simulink library "Power_Shaft1_FuelCell_A1"  (R2025b)
settings: Solver=VariableStepAuto  StartTime=0.0  StopTime=10.0  RelTol=1e-3
undefined symbols (not defined in the file): Init, Powertrain
libraries: fl_lib x85, nesl_utility x30, GasN_lib x21, simulink_extras x6, SimscapeFluids_lib x6, customMath_lib x5, ee_lib x3, slpidlib x3, gn_supplement_lib x2, batteryecm_lib x1, simulink x1, sm_lib x1
(part 3 of 3)

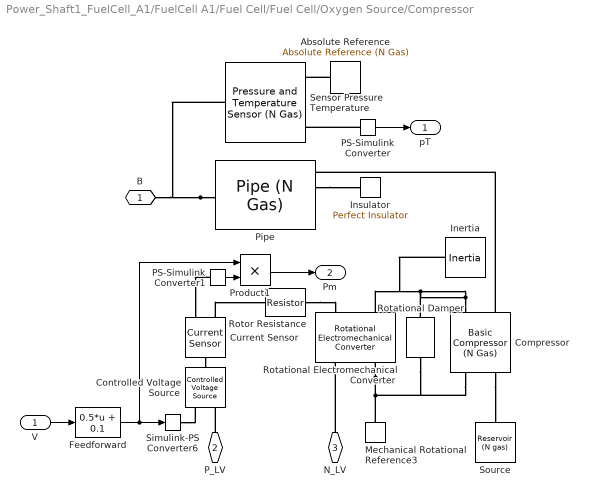
== system Power_Shaft1_FuelCell_A1/FuelCell A1/Fuel Cell/Fuel Cell/Oxygen Source/Compressor ==
  V : Inport
  Absolute Reference : GasN_lib/Absolute Reference (N Gas)
      settings: InternalSimscapePortConfiguration="{\"Bottom\":[],\"Left\":[{\"id\":\"A\",\"label\":\"\",\"type\":\"GasN.GasN\"}],\"Right\":[],\"Top\":[]}"
  Compressor : GasN_lib/Basic Compressor (N Gas)  pr_des=FuelCell.Compressor.rPressure.Value  mdot_corr_des=FuelCell.Compressor.mdotDesign.Value kg/s  omega_corr_des=FuelCell.Compressor.wDesign.Value rad/s  p_ref=FuelCell.Compressor.pReference.Value MPa  T_ref=FuelCell.Compressor.TReference.Value K  RH_ref=FuelCell.Compressor.relHumidity.Value  b1=FuelCell.Compressor.kSpeedCurve.Value  b2=FuelCell.Compressor.kSpeedOffset.Value  b3=FuelCell.Compressor.kSpeedSharp.Value  eta_poly=FuelCell.Compressor.effPolytropic.Value  eta_mech=FuelCell.Compressor.effMechanical.Value  area_A=FuelCell.Compressor.areaInlet.Value cm^2  area_B=FuelCell.Compressor.areaOutlet.Value cm^2  mdot_A_specify=off  mdot_A_priority=None  mdot_A=0.1 kg/s  mdot_A_nominal_specify=off  mdot_A_nominal_value=1  mdot_A_nominal_unit=kg/s  mdot_B_specify=off  mdot_B_priority=None  mdot_B=0.1 kg/s  mdot_B_nominal_specify=off  mdot_B_nominal_value=1  mdot_B_nominal_unit=kg/s  Phi_A_specify=off  Phi_A_priority=None  Phi_A=0 J/s  Phi_A_nominal_specify=off  Phi_A_nominal_value=1  Phi_A_nominal_unit=J/s  Phi_B_specify=off  Phi_B_priority=None  Phi_B=0 J/s  Phi_B_nominal_specify=off  Phi_B_nominal_value=1  Phi_B_nominal_unit=J/s  mdot_A_i_specify=off  mdot_A_i_priority=None  mdot_A_i=[ 0; 0; 0; 0 ] kg/s  mdot_A_i_nominal_specify=off  mdot_A_i_nominal_value=1  mdot_A_i_nominal_unit=kg/s  mdot_B_i_specify=off  mdot_B_i_priority=None  mdot_B_i=[ 0; 0; 0; 0 ] kg/s  mdot_B_i_nominal_specify=off  mdot_B_i_nominal_value=1  mdot_B_i_nominal_unit=kg/s  torque_specify=off  torque_priority=None  torque=1 N*m  torque_nominal_specify=off  torque_nominal_value=1  torque_nominal_unit=N*m
      settings: InternalSimscapePortConfiguration="{\"Bottom\":[],\"Left\":[{\"id\":\"A\",\"label\":\"A\",\"type\":\"GasN.GasN\"},{\"id\":\"Case\",\"label\":\"C\",\"type\":\"foundation.mechanical.rotational.rotational\"}],\"Right\":[{\"id\":\"B\",\"label\":\"B\",\"type\":\"GasN.GasN\"},{\"id\":\"Rod\",\"label\":\"R\",\"type\":\"foundation.mechanical.rotational.rotational\"}],\"Top\":[]}"
  Controlled Voltage Source : fl_lib/Electrical/Electrical Sources/Controlled Voltage Source
  Current Sensor : fl_lib/Electrical/Electrical Sensors/Current Sensor
  Feedforward : Fcn  Expr=0.5*u + 0.1
  Inertia : fl_lib/Mechanical/Rotational Elements/Inertia  inertia=FuelCell.Compressor.J.Value kg*m^2  num_ports=foundation.enum.numPorts2.one  w_specify=on  w_priority=High  w=0 rad/s  w_nominal_specify=off  w_nominal_value=1  w_nominal_unit=rad/s  t_specify=off  t_priority=None  t=0 N*m  t_nominal_specify=off  t_nominal_value=1  t_nominal_unit=N*m
  Insulator : fl_lib/Thermal/Thermal Elements/Perfect Insulator  T_specify=off  T_priority=None  T=0 K  T_nominal_specify=off  T_nominal_value=1  T_nominal_unit=K
  Mechanical Rotational Reference3 : fl_lib/Mechanical/Rotational Elements/Mechanical Rotational Reference
  PS-Simulink Converter : nesl_utility/PS-Simulink Converter  PhysicalDomain=network_engine_domain  SubClassName=ps_output  LeftPortType=input  RightPortType=output  PseudoPeriodic=off  Frequencies=[]  VectorFormat=1-D array  Unit=Pa  AffineConversion=off
  PS-Simulink Converter1 : nesl_utility/PS-Simulink Converter  PhysicalDomain=network_engine_domain  SubClassName=ps_output  LeftPortType=input  RightPortType=output  PseudoPeriodic=off  Frequencies=[]  VectorFormat=1-D array  Unit=A  AffineConversion=off
  Pipe : GasN_lib/Pipe (N Gas)  length=FuelCell.CompressorPipe.xPipe.Value m  area=FuelCell.CompressorPipe.areaPipe.Value cm^2  Dh=FuelCell.CompressorPipe.dHydraulic.Value cm  extra_length=FuelCell.CompressorPipe.xFriction.Value m  roughness=FuelCell.CompressorPipe.roughness.Value m  Re_lam=FuelCell.CompressorPipe.laminarReynoldsMax.Value  Re_tur=FuelCell.CompressorPipe.turbulentReynoldsMin.Value  shape_factor=FuelCell.CompressorPipe.frictionDarcy.Value  Nu_lam=FuelCell.CompressorPipe.laminarNusselt.Value  p0=FuelCell.CompressorPipe.p.Value MPa  T0=FuelCell.CompressorPipe.T.Value degC  comp=GasN.composition_enum.mole  y0=FuelCell.CompressorPipe.rMoleFractions.Value'  x0=[1; 0; 0; 0]  tau_c=FuelCell.CompressorPipe.timeCondensation.Value s  isCond=FuelCell.CompressorPipe.speciesCondensed.Value'
      settings: InternalSimscapePortConfiguration="{\"Bottom\":[],\"Left\":[{\"id\":\"A\",\"label\":\"A\",\"type\":\"GasN.GasN\"},{\"id\":\"H\",\"label\":\"H\",\"type\":\"foundation.thermal.thermal\"},{\"id\":\"MIn\",\"label\":\"M_in\",\"type\":\"input\"},{\"id\":\"TIn\",\"label\":\"T_in\",\"type\":\"input\"}],\"Right\":[{\"id\":\"B\",\"label\":\"B\",\"type\":\"GasN.GasN\"}],\"Top\":[]}"
  Product1 : Product
  Rotational Electromechanical Converter : fl_lib/Electrical/Electrical Elements/Rotational Electromechanical Converter  K=FuelCell.Compressor.KMotor.Value V/(rad/s)  i_specify=off  i_priority=None  i=0 A  i_nominal_specify=off  i_nominal_value=1  i_nominal_unit=A  v_specify=off  v_priority=None  v=0 V  v_nominal_specify=off  v_nominal_value=1  v_nominal_unit=V  t_specify=off  t_priority=None  t=0 N*m  t_nominal_specify=off  t_nominal_value=1  t_nominal_unit=N*m  w_specify=off  w_priority=None  w=0 rad/s  w_nominal_specify=off  w_nominal_value=1  w_nominal_unit=rad/s
  Rotational Damper : fl_lib/Mechanical/Rotational Elements/Rotational Damper  D=FuelCell.Compressor.b.Value N*m/(rad/s)  w_specify=off  w_priority=None  w=0 rad/s  w_nominal_specify=off  w_nominal_value=1  w_nominal_unit=rad/s  t_specify=off  t_priority=None  t=0 N*m  t_nominal_specify=off  t_nominal_value=1  t_nominal_unit=N*m
  Rotor Resistance : fl_lib/Electrical/Electrical Elements/Resistor  Tag=Factory Generic  R=FuelCell.Compressor.rMotor.Value Ohm  i_specify=off  i_priority=High  i=0 A  i_nominal_specify=off  i_nominal_value=1  i_nominal_unit=A  v_specify=off  v_priority=High  v=0 V  v_nominal_specify=off  v_nominal_value=1  v_nominal_unit=V
  Sensor Pressure Temperature : GasN_lib/Pressure and Temperature Sensor (N Gas)
      settings: InternalSimscapePortConfiguration="{\"Bottom\":[],\"Left\":[{\"id\":\"A\",\"label\":\"A\",\"type\":\"GasN.GasN\"}],\"Right\":[{\"id\":\"p\",\"label\":\"p\",\"type\":\"output\"},{\"id\":\"T\",\"label\":\"T\",\"type\":\"output\"},{\"id\":\"B\",\"label\":\"B\",\"type\":\"GasN.GasN\"}],\"Top\":[]}"
  Simulink-PS Converter6 : nesl_utility/Simulink-PS Converter  PhysicalDomain=network_engine_domain  SubClassName=ps_input  LeftPortType=input  RightPortType=output  PseudoPeriodic=off  Frequencies=[]  NoiseDistribution=none  NoiseParameters=[]  Unit=V  AffineConversion=off  FilteringAndDerivatives=filter  SimscapeFilterOrder=1  InputFilterTimeConstant=0.01  UdotUserProvided=0
  Source : GasN_lib/Reservoir (N gas)  p0=FuelCell.CompressorSource.p.Value MPa  T0=FuelCell.CompressorSource.T.Value degC  constCond=true  comp=GasN.composition_enum.mole  y0=FuelCell.CompressorSource.rMoleFractions.Value'  x0=[1; 0; 0; 0]  area=FuelCell.CompressorSource.areaPipe.Value cm^2
      settings: InternalSimscapePortConfiguration="{\"Bottom\":[],\"Left\":[{\"id\":\"A\",\"label\":\"A\",\"type\":\"GasN.GasN\"}],\"Right\":[],\"Top\":[]}"
  B : PMIOPort  Side=Left
  P_LV : PMIOPort  Port=2  Side=Right
  N_LV : PMIOPort  Port=3  Side=Right
  pT : Outport
  Pm : Outport  Port=2
  wires:
  Feedforward/1 -> Simulink-PS Converter6/1, Product1/1
  PS-Simulink Converter1/1 -> Product1/2
  Product1/1 -> Pm/1
  PS-Simulink Converter/1 -> pT/1
  V/1 -> Feedforward/1
  connections:
  Pipe/LConn2 -- Insulator/LConn1
  Rotor Resistance/RConn1 -- Rotational Electromechanical Converter/LConn1
  PS-Simulink Converter1/LConn1 -- Current Sensor/RConn1
  Compressor/LConn1 -- Source/LConn1
  Compressor/RConn1 -- Pipe/LConn1
  PS-Simulink Converter/LConn1 -- Sensor Pressure Temperature/RConn1
  Absolute Reference/LConn1 -- Sensor Pressure Temperature/RConn3
  Pipe/RConn1 -- Sensor Pressure Temperature/LConn1 -- B/RConn1
  Current Sensor/RConn2 -- Rotor Resistance/LConn1
  Current Sensor/LConn1 -- Controlled Voltage Source/LConn1
  Rotational Electromechanical Converter/RConn2 -- Rotational Damper/RConn1 -- Compressor/LConn2 -- Mechanical Rotational Reference3/LConn1
  N_LV/RConn1 -- Rotational Electromechanical Converter/RConn1
  P_LV/RConn1 -- Controlled Voltage Source/RConn2
  Simulink-PS Converter6/RConn1 -- Controlled Voltage Source/RConn1
  Compressor/RConn2 -- Inertia/LConn1 -- Rotational Electromechanical Converter/LConn2 -- Rotational Damper/LConn1

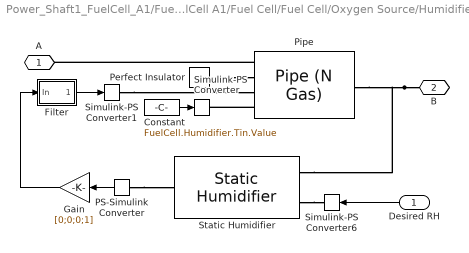
== system Power_Shaft1_FuelCell_A1/FuelCell A1/Fuel Cell/Fuel Cell/Oxygen Source/Humidifier ==
  Desired RH : Inport
  Constant : Constant  Value=FuelCell.Humidifier.Tin.Value
  Filter : Subsystem  mask(First-order lag supporting vector signals){b=[1 1 1 1]*0.01, x_initial=[0 0 0 0]}
      mask prompts: b "Filter time constant"; x_initial "Initial output"
      mask help: Models a lag of the form 1/(b*s+1) where s is the Laplace operator.
  Gain : Gain  Gain=[0;0;0;1]
  PS-Simulink Converter : nesl_utility/PS-Simulink Converter  PhysicalDomain=network_engine_domain  SubClassName=ps_output  LeftPortType=input  RightPortType=output  PseudoPeriodic=off  Frequencies=[]  VectorFormat=1-D array  Unit=1  AffineConversion=off
  Perfect Insulator : fl_lib/Thermal/Thermal Elements/Perfect Insulator  T_specify=off  T_priority=None  T=0 K  T_nominal_specify=off  T_nominal_value=1  T_nominal_unit=K
  Pipe : GasN_lib/Pipe (N Gas)  length=FuelCell.Humidifier.xPipe.Value m  area=FuelCell.Humidifier.areaPipe.Value cm^2  Dh=FuelCell.Humidifier.dHydraulic.Value cm  extra_length=FuelCell.Humidifier.xFriction.Value m  roughness=FuelCell.Humidifier.roughness.Value m  Re_lam=FuelCell.Humidifier.laminarReynoldsMax.Value  Re_tur=FuelCell.Humidifier.turbulentReynoldsMin.Value  shape_factor=FuelCell.Humidifier.frictionDarcy.Value  Nu_lam=FuelCell.Humidifier.laminarNusselt.Value  p0=FuelCell.Humidifier.p.Value MPa  T0=FuelCell.Humidifier.T.Value degC  comp=GasN.composition_enum.mole  y0=FuelCell.Humidifier.rMoleFractions.Value'  x0=[1; 0; 0; 0]  tau_c=FuelCell.Humidifier.timeCondensation.Value s  isCond=FuelCell.Humidifier.speciesCondensed.Value'
      settings: InternalSimscapePortConfiguration="{\"Bottom\":[],\"Left\":[{\"id\":\"A\",\"label\":\"A\",\"type\":\"GasN.GasN\"},{\"id\":\"H\",\"label\":\"H\",\"type\":\"foundation.thermal.thermal\"},{\"id\":\"MIn\",\"label\":\"M_in\",\"type\":\"input\"},{\"id\":\"TIn\",\"label\":\"T_in\",\"type\":\"input\"}],\"Right\":[{\"id\":\"B\",\"label\":\"B\",\"type\":\"GasN.GasN\"}],\"Top\":[]}"
  Simulink-PS Converter : nesl_utility/Simulink-PS Converter  PhysicalDomain=network_engine_domain  SubClassName=ps_input  LeftPortType=input  RightPortType=output  PseudoPeriodic=off  Frequencies=[]  NoiseDistribution=none  NoiseParameters=[]  Unit=1  AffineConversion=off  FilteringAndDerivatives=provide  SimscapeFilterOrder=1  InputFilterTimeConstant=0.001  UdotUserProvided=0
  Simulink-PS Converter1 : nesl_utility/Simulink-PS Converter  PhysicalDomain=network_engine_domain  SubClassName=ps_input  LeftPortType=input  RightPortType=output  PseudoPeriodic=off  Frequencies=[]  NoiseDistribution=none  NoiseParameters=[]  Unit=1  AffineConversion=off  FilteringAndDerivatives=provide  SimscapeFilterOrder=1  InputFilterTimeConstant=0.001  UdotUserProvided=0
  Simulink-PS Converter6 : nesl_utility/Simulink-PS Converter  PhysicalDomain=network_engine_domain  SubClassName=ps_input  LeftPortType=input  RightPortType=output  PseudoPeriodic=off  Frequencies=[]  NoiseDistribution=none  NoiseParameters=[]  Unit=1  AffineConversion=off  FilteringAndDerivatives=provide  SimscapeFilterOrder=1  InputFilterTimeConstant=0.001  UdotUserProvided=0
  Static Humidifier : gn_supplement_lib/Static Humidifier  Kp=0.5 kg/s
      settings: InternalSimscapePortConfiguration="{\"Bottom\":[],\"Left\":[{\"id\":\"Rh_des\",\"label\":\"Rh_des\",\"type\":\"input\"},{\"id\":\"A\",\"label\":\"A\",\"type\":\"GasN.GasN\"}],\"Right\":[{\"id\":\"m_add\",\"label\":\"m_add\",\"type\":\"output\"}],\"Top\":[]}"
  A : PMIOPort  Side=Left
  B : PMIOPort  Port=2  Side=Right
  wires:
  Filter/1(Out) -> Simulink-PS Converter1/1
  Gain/1 -> Filter/1(In)
  PS-Simulink Converter/1 -> Gain/1
  Constant/1 -> Simulink-PS Converter/1
  Desired RH/1 -> Simulink-PS Converter6/1
  connections:
  Perfect Insulator/LConn1 -- Pipe/LConn2
  Pipe/LConn4 -- Simulink-PS Converter/RConn1
  Simulink-PS Converter1/RConn1 -- Pipe/LConn3
  PS-Simulink Converter/LConn1 -- Static Humidifier/RConn1
  Static Humidifier/LConn1 -- Simulink-PS Converter6/RConn1
  Pipe/LConn1 -- A/RConn1
  B/RConn1 -- Static Humidifier/LConn2 -- Pipe/RConn1

== system Power_Shaft1_FuelCell_A1/FuelCell A1/Fuel Cell/Fuel Cell/ThermalMgmt/Pump Control ==
  TStack : Inport
  TRef : Inport  Port=2
  PID Controller : slpidlib/PID Controller  Controller=PID  Form=Parallel  TimeDomain=Continuous-time  UseExternalTs=off  SampleTime=-1  IntegratorMethod=Forward Euler  FilterMethod=Forward Euler  ControllerParametersSource=internal  P=FuelCell.Thermal.PumpCtrl.Kp.Value  I=FuelCell.Thermal.PumpCtrl.Ki.Value  UseKiTs=off  D=FuelCell.Thermal.PumpCtrl.Kd.Value  N=FuelCell.Thermal.PumpCtrl.filter.Value  UseFilter=on  TunerSelectOption=Transfer Function Based (PID Tuner App)  ZeroCross=off  InitialConditionSource=internal  InitialConditionForIntegrator=FuelCell.Thermal.PumpCtrl.lowerlim.Value  InitialConditionForFilter=FuelCell.Thermal.PumpCtrl.lowerlim.Value  DifferentiatorICPrevScaledInput=0  ExternalReset=none  TrackingMode=off  Kt=1  LimitOutput=on  SatLimitsSource=internal  UpperSaturationLimit=FuelCell.Thermal.PumpCtrl.upperlim.Value  LowerSaturationLimit=FuelCell.Thermal.PumpCtrl.lowerlim.Value  LinearizeAsGain=on  AntiWindupMode=clamping  Kb=1  POutMin=[]  POutMax=[]  IOutMin=[]  IOutMax=[]  DOutMin=[]  DOutMax=[]  NOutMin=[]  NOutMax=[]  SumOutMin=[]  SumOutMax=[]  SaturationOutMin=[]  SaturationOutMax=[]  PParamMin=[]  PParamMax=[]  IParamMin=[]  IParamMax=[]  DParamMin=[]  DParamMax=[]  NParamMin=[]  NParamMax=[]  KbParamMin=[]  KbParamMax=[]  KtParamMin=[]  KtParamMax=[]  KbOutMin=[]  KbOutMax=[]  KtOutMin=[]  KtOutMax=[]  IntegratorOutMin=[]  IntegratorOutMax=[]  FilterOutMin=[]  FilterOutMax=[]  SumI1OutMin=[]  SumI1OutMax=[]  SumI2OutMin=[]  SumI2OutMax=[]  SumI3OutMin=[]  SumI3OutMax=[]  SumI4OutMin=[]  SumI4OutMax=[]  SumDOutMin=[]  SumDOutMax=[]  DifferentiatorOutMin=[]  DifferentiatorOutMax=[]  FilterDiffOutCoefMin=[]  FilterDiffOutCoefMax=[]  ReciprocalOutMin=[]  ReciprocalOutMax=[]  SumDenOutMin=[]  SumDenOutMax=[]  SumNumOutMin=[]  SumNumOutMax=[]  DivideOutMin=[]  DivideOutMax=[]  UdiffTsProdOutMin=[]  UdiffTsProdOutMax=[]  NTsProdOutMin=[]  NTsProdOutMax=[]  UintegralTsProdOutMin=[]  UintegralTsProdOutMax=[]  UngainTsProdOutMin=[]  UngainTsProdOutMax=[]  IntegratorContinuousStateAttributes=''  IntegratorStateMustResolveToSignalObject=off  IntegratorRTWStateStorageClass=Auto  FilterContinuousStateAttributes=''  FilterStateMustResolveToSignalObject=off  FilterRTWStateStorageClass=Auto  ParallelPVariant=InternalParameters  IdealPVariant=Disabled  IVariant=InternalParameters  DVariant=InternalParameters  IntegratorVariant=Continuous  SatVariant=Enabled  AWVariant=ContClampingParallel  PCopyVariant=Disabled  TRVariant=Disabled  FdbkBlocksVariant=Forward  IdealPFdbkVariant=Disabled  SatFdbkVariant=Disabled  DerivativeFilterVariant=ContFilter  NVariant=InternalParameters  NCopyVariant=Disabled  FilterICVariant=InternalICsFilter  IntegratorICVariant=InternalICs  ExternalResetVariant=Disabled  TRSumVariant=Passthrough  SumFdbkVariant=Disabled  SumVariant=Sum_PID  TsampFilterVariant=InternalTs  TsampNgainVariant=Passthrough  TsampIntegralVariant=Passthrough  ExternalSaturationOutDataTypeStr=Inherit: Same as second input
  Subtract : Sum  Inputs=+-
  Transfer Fcn (with initial outputs)1 : simulink_extras/Additional Linear/Transfer Fcn (with initial outputs)  N=[1]  D="[1  1]"  Y0=.5  U0=80
  y : Outport
  wires:
  TStack/1 -> Subtract/2
  PID Controller/1 -> y/1
  TRef/1 -> Transfer Fcn (with initial outputs)1/1
  Transfer Fcn (with initial outputs)1/1 -> Subtract/1
  Subtract/1 -> PID Controller/1

== system Power_Shaft1_FuelCell_A1/FuelCell A1/Fuel Cell/Fuel Cell/ThermalMgmt/Sensor TStack ==
  PS-Simulink Converter2 : nesl_utility/PS-Simulink Converter  PhysicalDomain=network_engine_domain  SubClassName=ps_output  LeftPortType=input  RightPortType=output  PseudoPeriodic=off  Frequencies=[]  VectorFormat=1-D array  Unit=degC  AffineConversion=on
  Temperature Sensor : fl_lib/Thermal/Thermal Sensors/Temperature Sensor  temperature_measure=foundation.enum.MeasurementReference.difference
  Thermal Reference : fl_lib/Thermal/Thermal Elements/Thermal Reference
  A : PMIOPort  Side=Left
  T : Outport
  wires:
  PS-Simulink Converter2/1 -> T/1
  connections:
  Temperature Sensor/LConn1 -- A/RConn1
  PS-Simulink Converter2/LConn1 -- Temperature Sensor/RConn2
  Thermal Reference/LConn1 -- Temperature Sensor/RConn1

== system Power_Shaft1_FuelCell_A1/FuelCell A1/Fuel Cell/Fuel Cell/ThermalMgmt/Tank ==
  Perfect Insulator : fl_lib/Thermal/Thermal Elements/Perfect Insulator  T_specify=off  T_priority=None  T=0 K  T_nominal_specify=off  T_nominal_value=1  T_nominal_unit=K
  Tank : SimscapeFluids_lib/Thermal Liquid/Tanks & Accumulators/Tank (TL)  num_inlet=2  pressure_spec=1  tank_pressure=0.101325 MPa  volume_spec=1  tank_area=FuelCell.Thermal.Tank.area.Value cm^2  level_TLU=[0, 3, 5] m  volume_TLU=[0, 4, 6] m^3  inlet_height_A=[.1] m  inlet_area_A=[.01] m^2  inlet_heights_AB=FuelCell.Thermal.Tank.elevationAB.Value m  inlet_areas_AB=FuelCell.Thermal.Tank.areaAB.Value cm^2  inlet_heights_ABC=[.1, .05, 0] m  inlet_areas_ABC=[.01, .01, .01] m^2  inlet_heights_ABCD=linspace(0.1, 0, 4) m  inlet_areas_ABCD=0.01 * ones(1, 4) m^2  inlet_heights_ABCDE=linspace(0.1, 0, 5) m  inlet_areas_ABCDE=0.01 * ones(1, 5) m^2  inlet_heights_ABCDEF=linspace(0.1, 0, 6) m  inlet_areas_ABCDEF=0.01 * ones(1, 6) m^2  level_check=simscape.enum.assert.action.error  capacity_check=1  max_capacity=FuelCell.Thermal.Tank.volume.Value l  g=FuelCell.Thermal.Tank.g.Value m/s^2  level_specify=on  level_priority=None  level=0 m  level_nominal_specify=off  level_nominal_value=1  level_nominal_unit=m  volume_specify=on  volume_priority=High  volume=FuelCell.Thermal.Tank.volumeLiquid.Value l  volume_nominal_specify=off  volume_nominal_value=1  volume_nominal_unit=m^3  mass_specify=off  mass_priority=None  mass=5e+3 kg  mass_nominal_specify=off  mass_nominal_value=1  mass_nominal_unit=kg  T_I_specify=off  T_I_priority=High  T_I=293.15 K  T_I_nominal_specify=off  T_I_nominal_value=1  T_I_nominal_unit=K
      settings: InternalSimscapePortConfiguration="{\"Bottom\":[{\"id\":\"H\",\"label\":\"H\",\"type\":\"foundation.thermal.thermal\"},{\"id\":\"T_out\",\"label\":\"T\",\"type\":\"output\"}],\"Left\":[{\"id\":\"A\",\"label\":\"A\",\"type\":\"foundation.thermal_liquid.thermal_liquid\"},{\"id\":\"B\",\"label\":\"B\",\"type\":\"foundation.thermal_liquid.thermal_liquid\"}],\"Right\":[],\"Top\":[{\"id\":\"V_out\",\"label\":\"V\",\"type\":\"output\"},{\"id\":\"L_out\",\"label\":\"L\",\"type\":\"output\"}]}"
  A : PMIOPort  Side=Right
  B : PMIOPort  Port=2  Side=Left
  connections:
  B/RConn1 -- Tank/LConn2
  Tank/LConn1 -- A/RConn1
  Tank/RConn1 -- Perfect Insulator/LConn1

== system Power_Shaft1_FuelCell_A1/FuelCell A1/Fuel Cell/Fuel Cell/Oxygen Source/Chiller/Heat Control ==
  TDes : Inport
  Absolute Reference (N Gas) : GasN_lib/Absolute Reference (N Gas)
      settings: InternalSimscapePortConfiguration="{\"Bottom\":[],\"Left\":[{\"id\":\"A\",\"label\":\"\",\"type\":\"GasN.GasN\"}],\"Right\":[],\"Top\":[]}"
  PS Subtract : customMath_lib/PS Subtract
      settings: InternalSimscapePortConfiguration="{\"Bottom\":[],\"Left\":[{\"id\":\"I1\",\"label\":\"\",\"type\":\"input\"},{\"id\":\"I2\",\"label\":\"\",\"type\":\"input\"}],\"Right\":[{\"id\":\"O\",\"label\":\"\",\"type\":\"output\"}],\"Top\":[]}"
  Product M cp : customMath_lib/PS Custom Product
      settings: InternalSimscapePortConfiguration="{\"Bottom\":[],\"Left\":[{\"id\":\"I1\",\"label\":\"\",\"type\":\"input\"},{\"id\":\"I2\",\"label\":\"\",\"type\":\"input\"}],\"Right\":[{\"id\":\"O\",\"label\":\"\",\"type\":\"output\"}],\"Top\":[]}"
  Product Q : customMath_lib/PS Custom Product
      settings: InternalSimscapePortConfiguration="{\"Bottom\":[],\"Left\":[{\"id\":\"I1\",\"label\":\"\",\"type\":\"input\"},{\"id\":\"I2\",\"label\":\"\",\"type\":\"input\"}],\"Right\":[{\"id\":\"O\",\"label\":\"\",\"type\":\"output\"}],\"Top\":[]}"
  Sensor Mass Flow Rate : GasN_lib/Mass Flow Rate Sensor (N Gas)
      settings: InternalSimscapePortConfiguration="{\"Bottom\":[],\"Left\":[{\"id\":\"A\",\"label\":\"A\",\"type\":\"GasN.GasN\"}],\"Right\":[{\"id\":\"M\",\"label\":\"M\",\"type\":\"output\"},{\"id\":\"Phi_out\",\"label\":\"Phi\",\"type\":\"output\"},{\"id\":\"M_i\",\"label\":\"M_i\",\"type\":\"output\"},{\"id\":\"B\",\"label\":\"B\",\"type\":\"GasN.GasN\"}],\"Top\":[]}"
  Sensor P T : GasN_lib/Pressure and Temperature Sensor (N Gas)
      settings: InternalSimscapePortConfiguration="{\"Bottom\":[],\"Left\":[{\"id\":\"A\",\"label\":\"A\",\"type\":\"GasN.GasN\"}],\"Right\":[{\"id\":\"p\",\"label\":\"p\",\"type\":\"output\"},{\"id\":\"T\",\"label\":\"T\",\"type\":\"output\"},{\"id\":\"B\",\"label\":\"B\",\"type\":\"GasN.GasN\"}],\"Top\":[]}"
  Sensor Thermo : GasN_lib/Thermodynamic Properties Sensor (N Gas)
      settings: InternalSimscapePortConfiguration="{\"Bottom\":[],\"Left\":[{\"id\":\"A\",\"label\":\"A\",\"type\":\"GasN.GasN\"}],\"Right\":[{\"id\":\"H\",\"label\":\"h\",\"type\":\"output\"},{\"id\":\"RHO\",\"label\":\"rho\",\"type\":\"output\"},{\"id\":\"CP\",\"label\":\"cp\",\"type\":\"output\"},{\"id\":\"S\",\"label\":\"s\",\"type\":\"output\"}],\"Top\":[]}"
  Simulink-PS Converter4 : nesl_utility/Simulink-PS Converter  PhysicalDomain=network_engine_domain  SubClassName=ps_input  LeftPortType=input  RightPortType=output  PseudoPeriodic=off  Frequencies=[]  NoiseDistribution=none  NoiseParameters=[]  Unit=K  AffineConversion=off  FilteringAndDerivatives=provide  SimscapeFilterOrder=1  InputFilterTimeConstant=0.001  UdotUserProvided=0
  A : PMIOPort  Side=Left
  Q : PMIOPort  Port=2  Side=Right
  B : PMIOPort  Port=3  Side=Right
  wires:
  TDes/1 -> Simulink-PS Converter4/1
  connections:
  B/RConn1 -- Sensor Mass Flow Rate/RConn4
  Product Q/RConn1 -- Q/RConn1
  PS Subtract/LConn1 -- Simulink-PS Converter4/RConn1
  Absolute Reference (N Gas)/LConn1 -- Sensor P T/RConn3
  Product M cp/RConn1 -- Product Q/LConn1
  PS Subtract/RConn1 -- Product Q/LConn2
  Product M cp/LConn1 -- Sensor Mass Flow Rate/RConn1
  PS Subtract/LConn2 -- Sensor P T/RConn2
  Product M cp/LConn2 -- Sensor Thermo/RConn3
  Sensor Mass Flow Rate/LConn1 -- A/RConn1 -- Sensor Thermo/LConn1 -- Sensor P T/LConn1

== system Power_Shaft1_FuelCell_A1/FuelCell A1/Fuel Cell/Fuel Cell/Oxygen Source/Humidifier/Filter ==
  In : Inport
  Gain : Gain  Gain=1./b
  Integrator : Integrator  InitialCondition=x_initial.*b
  Sum : Sum  Inputs=|+-  InputSameDT=on  SaturateOnIntegerOverflow=on  OutDataTypeStr=Inherit: Same as first input
  Out : Outport  VectorParamsAs1DForOutWhenUnconnected=off
  wires:
  Sum/1 -> Integrator/1
  In/1 -> Sum/1
  Integrator/1 -> Gain/1
  Gain/1 -> Sum/2, Out/1
